simulink model "power_KundurTwoAreaSystem"  (R2023a)
settings: Solver=FixedStepDiscrete  StartTime=0.0  StopTime=5  MaxStep=1/60  RelTol=1e-4
PreLoadFcn:
  | Ts=50e-6;
  | Tctrl=2*Ts;
  | PSSMODEL=1;
undefined symbols (not defined in the file): D1, Delta
libraries: spsThreePhaseVIMeasurementLib x15, spsGenericPowerSystemStabilizerLib x8, spsLoadFlowBusLib x6, spsThreePhaseParallelRLCLoadLib x4, spsThreePhasePISectionLineLib x4, spsSynchronousMachinepuStandardLib x4, spsExcitationSystemLib x4, spsSteamTurbineandGovernorLib x4, spsThreePhaseSeriesRLCLoadLib x4, spsThreePhaseTransformerTwoWindingsLib x4, spsThreePhaseFaultLib x4, spsThreePhaseBreakerLib x2
(part 1 of 2)
settings Model: ARTEMISmethode_block_infos=$$__separator__$$  ExtModeTrigMode=oneshot  Creator=The MathWorks, Inc.  LastModifiedBy=LENOVO
settings SolverCC: AlgebraicLoopSolver=TrustRegion
settings DataIOCC: SaveOutput=off  SignalLogging=off  DSMLogging=off  SaveTime=off  ReturnWorkspaceOutputs=off  TimeSaveName=t  SignalLoggingName=sigsOut
settings OptimizationCC: BlockReduction=off  BooleanDataType=off  OptimizeBlockIOStorage=off  BufferReuse=off  ReuseModelBlockBuffer=off  GlobalBufferReuse=off  ExpressionFolding=off  ExpressionDepthLimit=2147483647  LocalBlockOutputs=off  InitFltsAndDblsToZero=on  LifeSpan=inf  OptimizeDataStoreBuffers=off  BusAssignmentInplaceUpdate=off
settings DebuggingCC: SaveWithParameterizedLinksMsg=none  SignalResolutionControl=TryResolveAllWithWarning  MultiTaskDSMMsg=warning  MultiTaskCondExecSysMsg=none  FcnCallInpInsideContextMsg=warning  UnconnectedInputMsg=warning  UnconnectedLineMsg=warning  StateNameClashWarn=warning  SFUnexpectedBacktrackingDiag=warning  SFNoUnconditionalDefaultTransitionDiag=warning  SFExecutionAtInitializationDiag=none  ArithmeticOperatorsInVariantConditions=warning
settings HardwareCC: ProdBitPerPointer=32  ProdBitPerSizeT=32  ProdBitPerPtrDiffT=32  ProdLargestAtomicFloat=None  ProdIntDivRoundTo=Undefined  ProdEndianess=Unspecified  ProdWordSize=32  ProdHWDeviceType=32-bit Generic  TargetBitPerPointer=64  TargetBitPerSizeT=64  TargetBitPerPtrDiffT=64  TargetLongLongMode=on  TargetIntDivRoundTo=Zero  TargetEndianess=LittleEndian  TargetWordSize=64  TargetHWDeviceType=MATLAB Host  ProdEqTarget=off
settings ModelReferenceCC: EnableRefExpFcnMdlSchedulingChecks=on  PropagateSignalLabelsOutOfModel=off
settings SFSimCC: SimUseLocalCustomCode=off  CustomCodeUndefinedFunction=UseInterfaceOnly
settings RTWCC: RTWUseLocalCustomCode=off
settings CodeAppCC: StateflowObjectComments=on
settings GRTTargetCC: TargetFcnLib=ansi_tfl_tmw.mat  TargetLangStandard=C89/C90 (ANSI)  CombineOutputUpdateFcns=off  GRTInterface=on
settings ConfigComp: CovMetricSettings=dw  CovSaveCumulativeToWorkspaceVar=on  CovSaveSingleToWorkspaceVar=on  CovExternalEMLEnable=off  CovSFcnEnable=off
settings SimscapeCC: SimscapeNormalizeSystem=off  SimscapeNominalValues={1, 'bar'; 1, 'cm^3/s'; 1, 'bar*kg/s'; 1, 'kJ/kg'; 1, 'kW'; }

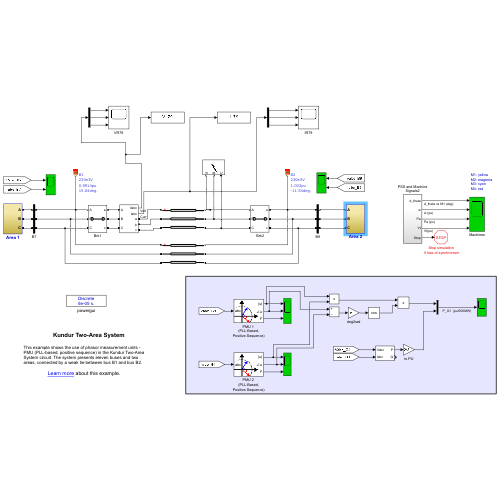
[thumbnail: Simulink's stored preview of the top-level diagram]
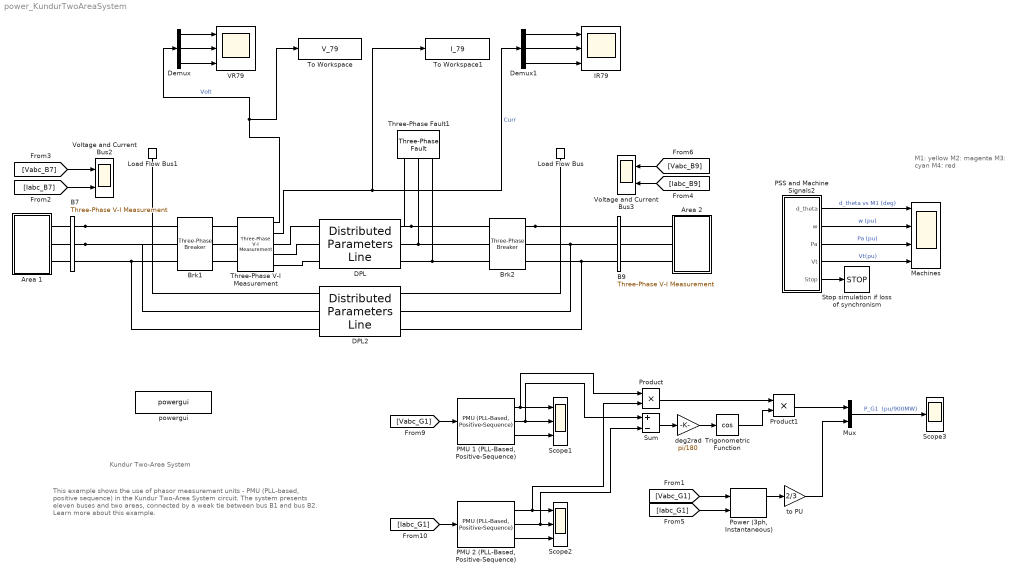
== system power_KundurTwoAreaSystem ==
  note: This example shows the use of phasor measurement units - PMU (PLL-based, positive sequence) in the Kundur Two-Area System circuit. The system presents eleven buses and two areas, connected by a weak tie between bus B1 and bus B2.
      |
      | Learn more about this example.
  note: M1: yellow
      | M2: magenta
      | M3: cyan
      | M4: red
  note: Kundur Two-Area System
  " Brk2" : spsThreePhaseBreakerLib/Three-Phase Breaker  InitialState=closed  SwitchA=on  SwitchB=on  SwitchC=on  SwitchTimes=[2+12]*100  External=off  BreakerResistance=0.001  SnubberResistance=1e6  SnubberCapacitance=0  Measurements=None
      settings: AttributesFormatString=\n
  Area 1 : Subsystem
  Area 2 : Subsystem
  B7 : spsThreePhaseVIMeasurementLib/Three-Phase V-I Measurement  VoltageMeasurement=phase-to-ground  SetLabelV=on  LabelV=Vabc_B7  Vpu=on  VpuLL=off  CurrentMeasurement=yes  SetLabelI=on  LabelI=Iabc_B7  Ipu=off  Pbase=100e6  Vbase=230e3  OutputType=Complex  PhasorSimulation=off  PSBequivalent=0
  B9 : spsThreePhaseVIMeasurementLib/Three-Phase V-I Measurement  VoltageMeasurement=phase-to-ground  SetLabelV=on  LabelV=Vabc_B9  Vpu=off  VpuLL=off  CurrentMeasurement=yes  SetLabelI=on  LabelI=Iabc_B9  Ipu=off  Pbase=100e6  Vbase=500e3  OutputType=Complex  PhasorSimulation=off  PSBequivalent=0
  Brk1 : spsThreePhaseBreakerLib/Three-Phase Breaker  InitialState=closed  SwitchA=off  SwitchB=off  SwitchC=off  SwitchTimes=[2+12]  External=off  BreakerResistance=0.001  SnubberResistance=inf  SnubberCapacitance=0  Measurements=None
      settings: AttributesFormatString=\n
  DPL : spsDistributedParametersLineLib/Distributed Parameters Line  Phases=3  Length=220  Frequency=60  Resistance=[0.0001*529 1.61]  Inductance=[0.001*529/(377) 0.0061]  Capacitance=[0.00175/529/(377) 5.2489e-9]  x1=[-0.00125 5.00367371114962e-05 67714.6934397594 -217896.109792038;-0.0012 4.86621318433669e-05 71809.6791282428 -216581.073841555;-0.00115 4.72702371515041e-05 75879.1511796623 -215189.087666813;-0.0011 4.58615475694642e-05 79921.6637299751 -213720.64583387;-0.00105 4.4436563597948e-05 83935.7804937212 -212176.270073119;-0.001 4.29957915269754e-05 87920.075274328 -210556.509093914;-0.00095 4.15397432560028e-05 91873.1324708315 -208861.938389617;-0.0009 4.00689361120477e-05 95793.547580833 -207093.160033131;-0.00085 3.8583892665885e-05 99679.9276995113 -205250.802462984;-0.0008 3.70851405463799e-05 103530.892014516 -203335.520260047;-0.00075 3.55732122530239e-05 107345.072296562 -201347.993914968;-0.0007 3.40486449667404e-05 111121.113385557 -199288.929586394;-0.00065 3.2511980359027e-05 114857.673672083 -197159.058850075;-0.0006 3.09637643995015e-05 118553.425574062 -194959.138438943;-0.00055 2.94045471619226e-05 122207.05600844 -192689.949974244;-0.0005 2.78348826287503e-05 125817.266857722 -190352.299687836;-0.00045 2.6255328494319e-05 129382.775431183 -187947.018135733;-0.0004 2.46664459666915e-05 132902.314920604 -185474.959903019;-0.00035 2.30687995682643e-05 136374.634850364 -182937.003300212;-0.0003 2.14629569351953e-05 139798.501521726 -180334.050051208;-0.00025 1.98494886157256e-05 143172.698451165 -177667.024972904;-0.0002 1.82289678674665e-05 146496.026802577 -174936.875646609;-0.00015 1.66019704537234e-05 149767.305813225 -172144.572081379;-0.0001 1.49690744389303e-05 152985.373213251 -169291.106369375;-5e-05 1.33308599832661e-05 156149.085638633 -166377.492333378]  x2=[-0.00125 6.6417563157089e-05 -37052.7419451155 -227701.023522909;-0.0012 6.59388164154627e-05 -32754.3455922343 -228358.945598922;-0.00115 6.54366419263393e-05 -28444.3117763279 -228935.732828921;-0.0011 6.49112181099238e-05 -24124.1718318883 -229431.180283151;-0.00105 6.43627316467963e-05 -19795.460684067 -229845.11193149;-0.001 6.37913774115854e-05 -15459.716303323 -230177.380705994;-0.00095 6.31973584037304e-05 -11118.4791589897 -230427.86855315;-0.0009 6.25808856753561e-05 -6773.29167195314 -230596.486475819;-0.00085 6.19421782562878e-05 -2425.69766663739 -230683.174564855;-0.0008 6.12814630762299e-05 1922.75817750908 -230687.902020394;-0.00075 6.059897488414e-05 6270.5308748305 -230610.667162792;-0.0007 5.98949561648229e-05 10616.07568239 -230451.497433227;-0.00065 5.91696570527773e-05 14957.8486488092 -230210.449383946;-0.0006 5.84233352433242e-05 19294.3071628271 -229887.608658174;-0.00055 5.76562559010488e-05 23623.9105013821 -229483.089959682;-0.0005 5.68686915655888e-05 27945.120377024 -228997.037012038;-0.00045 5.60609220548025e-05 32256.40148446 -228429.62250754;-0.0004 5.52332343653508e-05 36556.2220460412 -227781.04804586;-0.00035 5.43859225707287e-05 40843.0543559962 -227051.544062416;-0.0003 5.35192877167822e-05 45115.3753232175 -226241.369746499;-0.00025 5.26336377147484e-05 49371.6670124087 -225350.812949186;-0.0002 5.17292872318557e-05 53610.4171833994 -224380.190081066;-0.00015 5.08065575795247e-05 57830.1198284372 -223329.845999824;-0.0001 4.98657765992071e-05 62029.2757072648 -222200.153887709;-5e-05 4.89072785459056e-05 66206.3928797934 -220991.51511895]  x3=[-0.00125 5.67524045659529e-09 -83.9619667865334 325.434737438529;-0.0012 5.93441221514109e-09 -90.0809906089823 323.794335553023;-0.00115 6.19147550528425e-09 -96.1680090843992 322.03889108188;-0.0011 6.44633899366183e-09 -102.220859524104 320.169027726161;-0.00105 6.69891212848996e-09 -108.237391379156 318.185409839415;-0.001 6.9491051717365e-09 -114.215467004436 316.088742191629;-0.00095 7.19682923100451e-09 -120.15296241814 313.879769718837;-0.0009 7.44199629111529e-09 -126.04776805642 311.559277258439;-0.00085 7.68451924537978e-09 -131.8977895229 309.128089270358;-0.0008 7.92431192654714e-09 -137.70094833281 306.587069544109;-0.00075 8.16128913741954e-09 -143.455182651456 303.937120891901;-0.0007 8.39536668112235e-09 -149.158448026785 301.179184827873;-0.00065 8.6264613910189e-09 -154.808718115766 298.314241233575;-0.0006 8.85449116025912e-09 -160.40398540434 295.343308009826;-0.00055 9.07937497095181e-09 -165.942261920683 292.267440715053;-0.0005 9.30103292294984e-09 -171.421579941519 289.08773219026;-0.00045 9.51938626223831e-09 -176.839992691245 285.805312170745;-0.0004 9.73435740891549e-09 -182.195575033613 282.421346884711;-0.00035 9.94586998475657e-09 -187.486424155717 278.937038638912;-0.0003 1.01538488403505e-08 -192.710660244058 275.353625391476;-0.00025 1.03582200818002e-08 -197.866427152428 271.672380312068;-0.0002 1.05589110969767e-08 -202.951893061395 267.894611329534;-0.00015 1.0755850581318e-08 -207.965251129137 264.021660667207;-0.0001 1.0948968563163e-08 -212.904720133404 260.054904366015;-5e-05 1.11381964286123e-08 -217.768545104379 255.995751795585]  x4=[-0.00125 9.68464422615185e-08 -1.96836906133708 -1426.6168237965;-0.0012 9.56560270886339e-08 24.921520258627 -1426.40038533004;-0.00115 9.44316257848021e-08 51.80255508111 -1425.67715359865;-0.0011 9.31736733739763e-08 78.6651847024365 -1424.44738556312;-0.00105 9.18826168006582e-08 105.499864958212 -1422.71151815417;-0.001 9.05589147711008e-08 132.297061614318 -1420.47016811722;-0.00095 8.92030375903321e-08 159.04725375438 -1417.72413179328;-0.0009 8.78154669950584e-08 185.740937162506 -1414.47438483598;-0.00085 8.63966959825051e-08 212.368627700085 -1410.72208186493;-0.0008 8.49472286352572e-08 238.920864675461 -1406.46855605551;-0.00075 8.34675799421615e-08 265.388214205267 -1401.7153186652;-0.0007 8.19582756153531e-08 291.761272566243 -1396.46405849659;-0.00065 8.04198519034725e-08 318.030669536333 -1390.71664129743;-0.0006 7.88528554011392e-08 344.187071723876 -1384.47510909768;-0.00055 7.72578428547491e-08 370.221185883724 -1377.741679484;-0.0005 7.56353809646651e-08 396.123762219079 -1370.51874481189;-0.00045 7.39860461838711e-08 421.885597667908 -1362.80887135563;-0.0004 7.23104245131612e-08 447.497539172743 -1354.61479839655;-0.00035 7.06091112929365e-08 472.950486932723 -1345.93943724976;-0.0003 6.88827109916829e-08 498.235397636705 -1336.78587022977;-0.00025 6.71318369912072e-08 523.343287676313 -1327.15734955535;-0.0002 6.53571113687047e-08 548.26523633777 -1317.05729619404;-0.00015 6.35591646757385e-08 572.992388971387 -1306.48929864672;-0.0001 6.17386357142074e-08 597.515960137573 -1295.4571116726;-5e-05 5.98961713093829e-08 621.827236728265 -1283.96465495517]  x5=0.00124486354111605  V1=ones(3,3)  V2=ones(3,3)  I1=ones(3,3)  I2=ones(3,3)  nHarmo=1  Measurements=None  Decoupling=off  VsMag0=0  VrMag0=0  VsAngle0=0  VrAngle0=0  IsMag0=0  IrMag0=0  IsAngle0=0  IrAngle0=0
      settings: LibrarySourceBlock=sps_lib/Power Grid Elements/Distributed Parameters Line
  DPL2 : spsDistributedParametersLineLib/Distributed Parameters Line  Phases=3  Length=220  Frequency=60  Resistance=[0.0001*529 1.61]  Inductance=[0.001*529/(377) 0.0061]  Capacitance=[0.00175/529/(377) 5.2489e-9]  x1=[-0.00125 5.00379847973649e-05 67714.9467441329 -217896.980956182;-0.0012 4.86633839020789e-05 71809.9488077379 -216581.940076482;-0.00115 4.72714931382089e-05 75879.437138463 -215189.948664753;-0.0011 4.58628070379157e-05 79921.9658664817 -213721.501288916;-0.00105 4.44378261006631e-05 83936.098700586 -212177.119681331;-0.001 4.29970566153929e-05 87920.4094384935 -210557.352553429;-0.00095 4.15410104806428e-05 91873.4824735709 -208862.775400759;-0.0009 4.00702050226714e-05 95793.913297792 -207093.990298514;-0.00085 3.85851628116544e-05 99680.3090007523 -205251.625687619;-0.0008 3.70864114760182e-05 103531.288764564 -203336.336151446;-0.00075 3.5574483514976e-05 107345.484354455 -201348.802183249;-0.0007 3.40499161093329e-05 111121.540604892 -199289.729944382;-0.00065 3.25132509306289e-05 114858.115901071 -197159.851013407;-0.0006 3.0965033948685e-05 118553.88265558 -194959.922126168;-0.00055 2.94058152376227e-05 122207.527780091 -192690.724906921;-0.0005 2.78361487804258e-05 125817.753151886 -190353.065590635;-0.00045 2.62565922721123e-05 129383.276075083 -187947.774736533;-0.0004 2.46677069215884e-05 132902.829736365 -185475.706933003;-0.00035 2.30700572522534e-05 136375.163655073 -182937.740493963;-0.0003 2.14642109014275e-05 139799.044127501 -180334.777146806;-0.00025 1.98507384186727e-05 143173.25466522 -177667.741712014;-0.0002 1.82302130630794e-05 146496.596427293 -174937.581774578;-0.00015 1.66032105995901e-05 149767.888646217 -172145.267347323;-0.0001 1.49703090944329e-05 152985.969047441 -169291.790526269;-5e-05 1.33320887097373e-05 156149.694262324 -166378.165138145]  x2=[-0.00125 6.64176958426058e-05 -37052.8319738182 -227700.14152326;-0.0012 6.59389266485741e-05 -32754.4522292874 -228358.065452929;-0.00115 6.54367296678802e-05 -28444.4349838437 -228934.854849298;-0.0011 6.49112833287199e-05 -24124.3115660918 -229430.304781838;-0.00105 6.43627743196758e-05 -19795.6168953113 -229844.239219549;-0.001 6.37913975233868e-05 -15459.888936107 -230176.511093496;-0.00095 6.3197355947308e-05 -11118.6681519778 -230427.002349064;-0.0009 6.25808606515828e-05 -6773.496957997 -230595.623987903;-0.00085 6.19421306740542e-05 -2425.91917279987 -230682.316099547;-0.0008 6.12813929524419e-05 1922.52052992806 -230687.047882702;-0.00075 6.05988822437122e-05 6270.277170266 -230609.817656188;-0.0007 5.98948410406701e-05 10615.806010982 -230450.652859537;-0.00065 5.91695194858025e-05 14957.5631063708 -230209.610043242;-0.0006 5.84231752824043e-05 19294.00585081 -229886.77484867;-0.00055 5.76560736030171e-05 23623.5935268411 -229482.261977626;-0.0005 5.68684869952149e-05 27944.7878525787 -228996.215151609;-0.00045 5.60606952847694e-05 32256.0535282547 -228428.807060741;-0.0004 5.52329854762288e-05 36555.8587817031 -227780.239302415;-0.00035 5.43856516509468e-05 40842.6759125913 -227050.742309668;-0.0003 5.3518994862597e-05 45114.9818352051 -226240.575269306;-0.00025 5.26333230302095e-05 49371.2586195931 -225350.026029823;-0.0002 5.17289508287692e-05 53609.9940308807 -224379.410999122;-0.00015 5.08061995774129e-05 57829.6820665593 -223329.075032102;-0.0001 4.98653971252664e-05 62028.8234915626 -222199.391308131;-5e-05 4.89068777349613e-05 66205.9263709369 -220990.761198457]  x3=[-0.00125 5.67701476718236e-09 -83.9470362519072 325.436899755658;-0.0012 5.93614409507095e-09 -90.0661034818627 323.796778902833;-0.00115 6.19316433922822e-09 -96.1531706541115 322.04161459626;-0.0011 6.44798418158524e-09 -102.206075062672 320.17203043746;-0.00105 6.70051308586539e-09 -108.222666139428 318.188690680783;-0.001 6.95066132975141e-09 -114.20080621822 316.0922999974;-0.00095 7.19834003676336e-09 -120.138371294344 313.883603224938;-0.0009 7.443461207836e-09 -126.0332517792 311.563385102845;-0.00085 7.68593775258441e-09 -131.88335324982 309.13246999357;-0.0008 7.92568352024683e-09 -137.686597193009 306.591721589677;-0.00075 8.16261333029358e-09 -143.440921743827 303.942042606977;-0.0007 8.39664300269133e-09 -149.14428241816 301.184374463793;-0.00065 8.62768938781182e-09 -154.794652839118 298.319696946488;-0.0006 8.85567039597459e-09 -160.390025456994 295.349027861342;-0.00055 9.08050502661299e-09 -165.928412262543 292.273422672937;-0.0005 9.30211339705333e-09 -171.407845493302 289.09397412915;-0.00045 9.5204167708968e-09 -176.826378332736 285.81181187291;-0.0004 9.73533758599417e-09 -182.182085601928 282.428102040838;-0.00035 9.94679948200319e-09 -187.473064443587 278.944046848926;-0.0003 1.01547273275191e-08 -192.697434998124 275.360884165393;-0.00025 1.03590472467685e-08 -197.853341071558 271.67988707088;-0.0002 1.05596866458569e-08 -202.938950795012 267.902363406126;-0.00015 1.07565742385613e-08 -207.952457275566 264.029655307303;-0.0001 1.09496400716574e-08 -212.89207923824 260.063138729157;-5e-05 1.1138815549774e-08 -217.756061658871 256.004222956143]  x4=[-0.00125 9.68461057473568e-08 -1.98289624558899 -1426.61901857765;-0.0012 9.56557230997411e-08 24.9070370221481 -1426.40285353559;-0.00115 9.44313544291841e-08 51.788120938229 -1425.67989435166;-0.0011 9.31734347480444e-08 78.6508047815356 -1424.45039788981;-0.00105 9.1882410989195e-08 105.485544368409 -1422.71480098428;-0.001 9.05587418472302e-08 132.282805443649 -1420.47372028438;-0.00095 8.92028976154931e-08 159.033067067996 -1417.72795203541;-0.0009 8.78153600189834e-08 185.726825000868 -1414.47847179577;-0.00085 8.63966220432021e-08 212.354595077178 -1410.72643409031;-0.0008 8.49471877589966e-08 238.906916577008 -1406.47317200015;-0.00075 8.34675721434664e-08 265.374355586962 -1401.72019668907;-0.0007 8.19583008969943e-08 291.747508351987 -1396.46919686656;-0.00065 8.04199102564676e-08 318.017004616485 -1390.72203818786;-0.0006 7.88529468047557e-08 344.173510953518 -1384.48076259108;-0.00055 7.72579672765117e-08 370.207734080932 -1377.74758757171;-0.0005 7.56355383603673e-08 396.110424163215 -1370.5249053948;-0.00045 7.3986236497591e-08 421.872378097919 -1362.81528224491;-0.0004 7.23106476772813e-08 447.484442785481 -1354.62145731444;-0.00035 7.06093672281675e-08 472.93751838127 -1345.94634183038;-0.0003 6.88829996070924e-08 498.222561528727 -1336.79301801995;-0.00025 6.71321581842514e-08 523.330588572417 -1327.16473801552;-0.0002 6.53574650252652e-08 548.252678749889 -1317.06492269912;-0.00015 6.35595506701629e-08 572.97997736117 -1306.49716048704;-0.0001 6.17390539093537e-08 597.503698914807 -1295.46520605489;-5e-05 5.98966215566684e-08 621.815130249304 -1283.97297900353]  x5=0.00124486354111605  V1=ones(3,3)  V2=ones(3,3)  I1=ones(3,3)  I2=ones(3,3)  nHarmo=1  Measurements=None  Decoupling=off  VsMag0=0  VrMag0=0  VsAngle0=0  VrAngle0=0  IsMag0=0  IrMag0=0  IsAngle0=0  IrAngle0=0
      settings: LibrarySourceBlock=sps_lib/Power Grid Elements/Distributed Parameters Line
  Demux : Demux  Outputs=3
  Demux1 : Demux  Outputs=3
  IR79 : Scope  NumInputPorts=3
  Load Flow Bus : spsLoadFlowBusLib/Load Flow Bus  LConnTagsString=a  Phases=single  Connectors=on one side  ID=B2  Vbase=230e3  Vref=1  Vangle=0  VLF=1.003  VLFb=1  VLFc=1  angleLF=-11.54  angleLFb=0  angleLFc=0
      settings: AttributesFormatString=%<ID>\n%<Vbase>V\n%<VLF>pu\n%<angleLF>deg.
  Load Flow Bus1 : spsLoadFlowBusLib/Load Flow Bus  LConnTagsString=a  Phases=single  Connectors=on one side  ID=B1  Vbase=230e3  Vref=1  Vangle=0  VLF=0.9914  VLFb=1  VLFc=1  angleLF=15.04  angleLFb=0  angleLFc=0
      settings: AttributesFormatString=%<ID>\n%<Vbase>V\n%<VLF>pu\n%<angleLF>deg.
  Machines : Scope  NumInputPorts=4
  Mux : Mux  Inputs=2
  "PMU 1 (PLL-Based, Positive-Sequence)" : spsPMUPLLBasedPositiveSequenceLib/PMU (PLL-Based, Positive-Sequence)  nominalFrequency=60  samplingRate=64  reportingFactor=1
      settings: LibrarySourceBlock=|
      | sps_lib/Sensors and Measurements/PMU
      | (PLL-Based,
      | Positive-Sequence)
  "PMU 2 (PLL-Based, Positive-Sequence)" : spsPMUPLLBasedPositiveSequenceLib/PMU (PLL-Based, Positive-Sequence)  nominalFrequency=60  samplingRate=64  reportingFactor=1
      settings: LibrarySourceBlock=|
      | sps_lib/Sensors and Measurements/PMU
      | (PLL-Based,
      | Positive-Sequence)
  PSS and Machine Signals2 : Subsystem
  "Power (3ph, Instantaneous)" : spsPower3phInstantaneousLib/Power (3ph, Instantaneous)
  Product : Product
  Product1 : Product
  Scope1 : Scope  NumInputPorts=3
  Scope2 : Scope  NumInputPorts=3
  Scope3 : Scope
  Stop simulation if loss of synchronism : Stop
  Sum : Sum  Inputs=+-
  Three-Phase V-I Measurement : spsThreePhaseVIMeasurementLib/Three-Phase V-I Measurement  VoltageMeasurement=phase-to-ground  SetLabelV=off  LabelV=Vabc  Vpu=off  VpuLL=off  CurrentMeasurement=yes  SetLabelI=off  LabelI=Iabc  Ipu=off  Pbase=100e6  Vbase=500e3  OutputType=Complex  PhasorSimulation=off  PSBequivalent=0
  Three-Phase Fault1 : spsThreePhaseFaultLib/Three-Phase Fault  InitialStates=0  FaultA=off  FaultB=off  FaultC=off  GroundFault=off  SwitchTimes=[0 0.1]  External=off  SwitchStatus=NaN  FaultResistance=0.001  GroundResistance=0.001  SnubberResistance=1e6  SnubberCapacitance=inf  Measurements=None
  To Workspace : ToWorkspace  VariableName=V_79  SampleTime=0.01
  To Workspace1 : ToWorkspace  VariableName=I_79  SampleTime=0.01
  Trigonometric Function : Trigonometry  Operator=cos
  VR79 : Scope  NumInputPorts=3
  Voltage and Current Bus2 : Scope  NumInputPorts=2
  Voltage and Current Bus3 : Scope  NumInputPorts=2
  deg2rad : Gain  Gain=pi/180
  powergui : spspowerguiLib/powergui  Priority=2  SimulationMode=Discrete  SampleTime=Ts  frequency=60  Iterations=50  frequencyindice=0  Pbase=100e6  ErrMax=1e-4  UnitsV=kV  UnitsW=MW  buscounter=0  FunctionMessages=off  echomessages=off  EnableUseOfTLC=off  CurrentSourceSwitches=off  DisableSnubberDevices=off  DisableRonSwitches=off  DisableVfSwitches=off  DisplayEquations=off  AutomaticDiscreteSolvers=off  SolverType=Tustin  Interpol=off  ExternalGateDelay=off  methode=off  Ts=0  x0status=blocks  SPID=off  SwTol=0  HookPort=off  NonlinearTolerance=1e-4  nMaxIteration=100  ContinueOnMaxIteration=off  RestoreLinks=warning  ResistiveCurrentMeasurement=off  Frange=logspace(0,3,50)  Ylog=off  Xlog=off  ShowGrid=off  save=off  variable=ZData  structure=0  ZoomFFT=on  StartTime=0.0  cycles=1  DisplayStyle=1  fundamental=60  FreqAxis=off  MaxFrequency=1000  frequencyindicesteady=1  RmsSteady=1  display=off
  to PU : Gain  Gain=2/3
  wires:
  [Iabc_B7] -> Voltage and Current Bus2/2
  [Vabc_B7] -> Voltage and Current Bus2/1
  [Iabc_B9] -> Voltage and Current Bus3/2
  [Vabc_B9] -> Voltage and Current Bus3/1
  PSS and Machine Signals2/1(d_theta) -> Machines/1  "d_theta vs M1 (deg)"
  PSS and Machine Signals2/2(w) -> Machines/2  "w (pu)"
  PSS and Machine Signals2/3(Pa) -> Machines/3  "Pa (pu)"
  PSS and Machine Signals2/4(Vt) -> Machines/4  "Vt(pu)"
  PSS and Machine Signals2/5(Stop) -> Stop simulation if loss of synchronism/1
  [Iabc_G1] -> "PMU 2 (PLL-Based, Positive-Sequence)"/1
  "PMU 2 (PLL-Based, Positive-Sequence)"/3 -> Scope2/3
  [Vabc_G1] -> "PMU 1 (PLL-Based, Positive-Sequence)"/1
  "PMU 1 (PLL-Based, Positive-Sequence)"/3 -> Scope1/3
  Product/1 -> Product1/1
  [Iabc_G1] -> "Power (3ph, Instantaneous)"/2
  "Power (3ph, Instantaneous)"/1 -> to PU/1
  "PMU 2 (PLL-Based, Positive-Sequence)"/1 -> Product/2, Scope2/1
  [Vabc_G1] -> "Power (3ph, Instantaneous)"/1
  "PMU 2 (PLL-Based, Positive-Sequence)"/2 -> Sum/2, Scope2/2
  deg2rad/1 -> Trigonometric Function/1
  "PMU 1 (PLL-Based, Positive-Sequence)"/1 -> Scope1/1, Product/1
  Trigonometric Function/1 -> Product1/2
  Product1/1 -> Mux/1
  Sum/1 -> deg2rad/1
  to PU/1 -> Mux/2
  "PMU 1 (PLL-Based, Positive-Sequence)"/2 -> Sum/1, Scope1/2
  Mux/1 -> Scope3/1  "P_G1  (pu/900MW)"
  Three-Phase V-I Measurement/1 -> To Workspace/1, Demux/1  "Volt"
  Three-Phase V-I Measurement/2 -> To Workspace1/1, Demux1/1  "Curr"
  Demux/1 -> VR79/1
  Demux/2 -> VR79/2
  Demux/3 -> VR79/3
  Demux1/1 -> IR79/1
  Demux1/2 -> IR79/2
  Demux1/3 -> IR79/3
  connections:
  " Brk2"/RConn1 -- DPL2/RConn1 -- B9/LConn1 -- Load Flow Bus/LConn1
  " Brk2"/RConn2 -- DPL2/RConn2 -- B9/LConn2
  " Brk2"/RConn3 -- DPL2/RConn3 -- B9/LConn3
  B9/RConn3 -- Area 2/LConn3
  B9/RConn2 -- Area 2/LConn2
  Area 2/LConn1 -- B9/RConn1
  Area 1/RConn3 -- B7/LConn3
  Area 1/RConn2 -- B7/LConn2
  Area 1/RConn1 -- B7/LConn1
  " Brk2"/LConn3 -- Three-Phase Fault1/LConn3 -- DPL/RConn3
  " Brk2"/LConn2 -- Three-Phase Fault1/LConn2 -- DPL/RConn2
  DPL/RConn1 -- " Brk2"/LConn1 -- Three-Phase Fault1/LConn1
  DPL2/LConn3 -- B7/RConn3 -- Brk1/LConn3
  B7/RConn2 -- DPL2/LConn2 -- Brk1/LConn2
  B7/RConn1 -- DPL2/LConn1 -- Brk1/LConn1 -- Load Flow Bus1/LConn1
  Three-Phase V-I Measurement/LConn1 -- Brk1/RConn1
  Three-Phase V-I Measurement/LConn2 -- Brk1/RConn2
  Three-Phase V-I Measurement/LConn3 -- Brk1/RConn3
  DPL/LConn1 -- Three-Phase V-I Measurement/RConn1
  DPL/LConn2 -- Three-Phase V-I Measurement/RConn2
  DPL/LConn3 -- Three-Phase V-I Measurement/RConn3

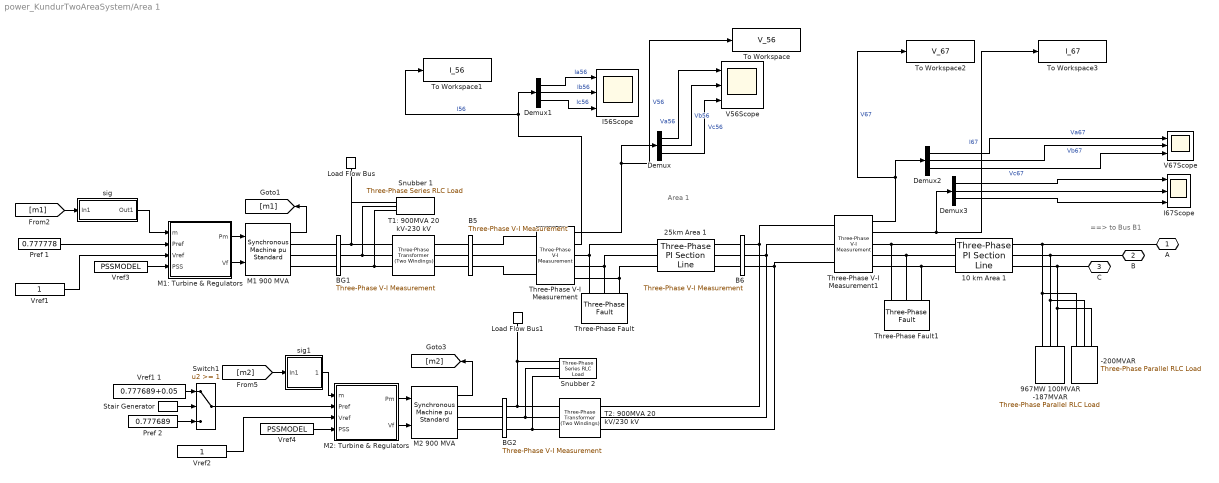
== system power_KundurTwoAreaSystem/Area 1 ==
  note: Area 1
  note: ==> to Bus B1
  -200MVAR : spsThreePhaseParallelRLCLoadLib/Three-Phase Parallel RLC Load  LConnTagsString=A|B|C  Configuration=Y (grounded)  NominalVoltage=230e3  Vabc=[1e3 1e3 1e3]  Vabcp=[1e3 1e3 1e3]  NominalFrequency=60  UnbalancedPower=off  ActivePower=0  InductivePower=0  CapacitivePower=200e6  Pabc=[10e3 9e3 11e3]  QLabc=[100 90 110]  QCabc=[100 90 110]  Pabcp=[10e3 9e3 11e3]  QLabcp=[100 90 110]  QCabcp=[100 90 110]  Measurements=None  LoadType=constant Z
  10 km Area 1 : spsThreePhasePISectionLineLib/Three-Phase PI Section Line  LConnTagsString=a|b|c  RConnTagsString=A|B|C  Length=10  Frequency=60  Resistances=[0.0001*529 1.61]  Inductances=[0.001*529/(377) 0.0061]  Capacitances=[0.00175/529/(377) 5.2489e-9]
  25km Area 1 : spsThreePhasePISectionLineLib/Three-Phase PI Section Line  LConnTagsString=a|b|c  RConnTagsString=A|B|C  Length=25  Frequency=60  Resistances=[0.0001*529 1.61]  Inductances=[0.001*529/(377) 0.0061]  Capacitances=[0.00175/529/(377) 5.2489e-9]
  967MW 100MVAR -187MVAR : spsThreePhaseParallelRLCLoadLib/Three-Phase Parallel RLC Load  LConnTagsString=A|B|C  Configuration=Y (grounded)  NominalVoltage=230e3  Vabc=[1e3 1e3 1e3]  Vabcp=[1e3 1e3 1e3]  NominalFrequency=60  UnbalancedPower=off  ActivePower=967e6  InductivePower=100e6  CapacitivePower=187e6  Pabc=[10e3 9e3 11e3]  QLabc=[100 90 110]  QCabc=[100 90 110]  Pabcp=[10e3 9e3 11e3]  QLabcp=[100 90 110]  QCabcp=[100 90 110]  Measurements=None  LoadType=constant Z
  B5 : spsThreePhaseVIMeasurementLib/Three-Phase V-I Measurement  VoltageMeasurement=phase-to-ground  SetLabelV=on  LabelV=Vabc_B5  Vpu=on  VpuLL=off  CurrentMeasurement=yes  SetLabelI=on  LabelI=Iabc_B5  Ipu=on  Pbase=900e6  Vbase=20e3  OutputType=Complex  PhasorSimulation=off  PSBequivalent=0
  B6 : spsThreePhaseVIMeasurementLib/Three-Phase V-I Measurement  VoltageMeasurement=phase-to-ground  SetLabelV=on  LabelV=Vabc_B6  Vpu=on  VpuLL=off  CurrentMeasurement=yes  SetLabelI=on  LabelI=Iabc_B6  Ipu=on  Pbase=900e6  Vbase=20e3  OutputType=Complex  PhasorSimulation=off  PSBequivalent=0
  BG1 : spsThreePhaseVIMeasurementLib/Three-Phase V-I Measurement  VoltageMeasurement=phase-to-ground  SetLabelV=on  LabelV=Vabc_G1  Vpu=on  VpuLL=off  CurrentMeasurement=yes  SetLabelI=on  LabelI=Iabc_G1  Ipu=on  Pbase=900e6  Vbase=20e3  OutputType=Complex  PhasorSimulation=off  PSBequivalent=0
  BG2 : spsThreePhaseVIMeasurementLib/Three-Phase V-I Measurement  VoltageMeasurement=no  SetLabelV=on  LabelV=Vabc_G2  Vpu=on  VpuLL=off  CurrentMeasurement=no  SetLabelI=on  LabelI=Iabc_G2  Ipu=on  Pbase=900e6  Vbase=20e3  OutputType=Complex  PhasorSimulation=off  PSBequivalent=0
  Demux{,1..3} (4 alike) : Demux  Outputs=3
  I56Scope : Scope  NumInputPorts=3
  I67Scope : Scope  NumInputPorts=3
  Load Flow Bus : spsLoadFlowBusLib/Load Flow Bus  LConnTagsString=a  Phases=single  Connectors=on one side  ID=M1_Area1  Vbase=20e3  Vref=1  Vangle=0  VLF=1  VLFb=1  VLFc=1  angleLF=10.19  angleLFb=0  angleLFc=0
      settings: AttributesFormatString=%<ID>\n%<Vbase>V\n%<VLF>pu\n%<angleLF>deg.
  Load Flow Bus1 : spsLoadFlowBusLib/Load Flow Bus  LConnTagsString=a  Phases=single  Connectors=on one side  ID=M2_Area1  Vbase=20e3  Vref=1  Vangle=0  VLF=1  VLFb=1  VLFc=1  angleLF=0  angleLFb=0  angleLFc=0
      settings: AttributesFormatString=%<ID>\n%<Vbase>V\n%<VLF>pu\n%<angleLF>deg.
  M1 900 MVA : spsSynchronousMachinepuStandardLib/Synchronous Machine pu Standard  PresetModel=No  MechanicalLoad=Mechanical power Pm  ShowDetailedParameters=on  RotorType=Round  Units=per unit standard parameters  MeasurementBus=off  NominalParameters="[900E6  20000   60 ]"  Reactances1=[1.8 .3 .25 1.7 .55 .25 .2]  Reactances2=[ 1.305, 0.296, 0.252, 0.474, 0.243, 0.18 ]  dAxisTimeConstants=Open-circuit  qAxisTimeConstants=Open-circuit  TimeConstants1=[]  TimeConstants2=[8 .03 .4 .05]  TimeConstants3=[]  TimeConstants4=[]  TimeConstants5=[ 1.01, 0.053, 0.1 ]  TimeConstants6=[]  TimeConstants7=[]  TimeConstants8=[]  StatorResistance=0.0025  Mechanical="[ 6.5 0  4]"  PolePairs=4  InitialConditions=[0 -31.4247 0.784453 0.784453 0.784453 2.7401 -117.26 122.74 1.83395]  SetSaturation=off  Saturation=[0.6404,0.7127,0.8441,0.9214,0.9956,1.082,1.19,1.316,1.457;0.7,0.7698,0.8872,0.9466,0.9969,1.046,1.1,1.151,1.201]  LoadFlowParameters=[1 700000000 0 0 0]  TsPowergui=0  TsBlock=-1  IterativeModel=Trapezoidal non iterative  IterativeDiscreteModel=Trapezoidal non iterative  BusType=PV  Pref=700000000  Qref=0  Qmin=-inf  Qmax=inf  PLF=0  QLF=0
  M1: Turbine & Regulators : Subsystem
  M2 900 MVA : spsSynchronousMachinepuStandardLib/Synchronous Machine pu Standard  PresetModel=No  MechanicalLoad=Mechanical power Pm  ShowDetailedParameters=on  RotorType=Round  Units=per unit standard parameters  MeasurementBus=off  NominalParameters="[900E6  20000   60 ]"  Reactances1=[1.8 .3 .25 1.7 .55 .25 .2]  Reactances2=[ 1.305, 0.296, 0.252, 0.474, 0.243, 0.18 ]  dAxisTimeConstants=Open-circuit  qAxisTimeConstants=Open-circuit  TimeConstants1=[]  TimeConstants2=[8 .03 .4 .05]  TimeConstants3=[]  TimeConstants4=[]  TimeConstants5=[ 1.01, 0.053, 0.1 ]  TimeConstants6=[]  TimeConstants7=[]  TimeConstants8=[]  StatorResistance=0.0025  Mechanical="[ 6.5 0  4]"  PolePairs=4  InitialConditions=[0 -42.8075 0.788608 0.788608 0.788608 -9.54571 -129.546 110.454 1.86756]  SetSaturation=off  Saturation=[0.6404,0.7127,0.8441,0.9214,0.9956,1.082,1.19,1.316,1.457;0.7,0.7698,0.8872,0.9466,0.9969,1.046,1.1,1.151,1.201]  LoadFlowParameters=[2 700000000 0 0 0]  TsPowergui=0  TsBlock=-1  IterativeModel=Trapezoidal non iterative  IterativeDiscreteModel=Trapezoidal non iterative  BusType=swing  Pref=0  Qref=0  Qmin=-inf  Qmax=inf  PLF=0  QLF=0
  M2: Turbine & Regulators : Subsystem
  Pref 1 : Constant  Value=0.777778
  Pref 2 : Constant  Value=0.777689
  Snubber 1 : spsThreePhaseSeriesRLCLoadLib/Three-Phase Series RLC Load  LConnTagsString=A|B|C  Configuration=Y (grounded)  NominalVoltage=20000  Vabc=[1e3 1e3 1e3]  Vabcp=[1e3 1e3 1e3]  NominalFrequency=60  UnbalancedPower=off  ActivePower=1e6  InductivePower=0  CapacitivePower=1e7  Pabc=[10e3 9e3 11e3]  QLabc=[100 90 110]  QCabc=[100 90 110]  Pabcp=[10e3 9e3 11e3]  QLabcp=[100 90 110]  QCabcp=[100 90 110]  Measurements=None  LoadType=constant Z
  Snubber 2 : spsThreePhaseSeriesRLCLoadLib/Three-Phase Series RLC Load  LConnTagsString=A|B|C  Configuration=Y (grounded)  NominalVoltage=20000  Vabc=[1e3 1e3 1e3]  Vabcp=[1e3 1e3 1e3]  NominalFrequency=60  UnbalancedPower=off  ActivePower=1e6  InductivePower=0  CapacitivePower=1e7  Pabc=[10e3 9e3 11e3]  QLabc=[100 90 110]  QCabc=[100 90 110]  Pabcp=[10e3 9e3 11e3]  QLabcp=[100 90 110]  QCabcp=[100 90 110]  Measurements=None  LoadType=constant Z
  Stair Generator : spsStairGeneratorLib/Stair Generator  t=[0 15 20]  e=[0 1 0 ]  Ts=0
  Switch1 : Switch  Threshold=1  SaturateOnIntegerOverflow=off
  T1: 900MVA 20 kV-230 kV : spsThreePhaseTransformerTwoWindingsLib/Three-Phase Transformer (Two Windings)  Winding1Connection=Delta (D1)  Winding2Connection=Yg  CoreType=Three single-phase transformers  SetSaturation=off  Hysteresis=off  DataFile='hysteresis'  SetInitialFlux=off  Measurements=None  UNITS=pu  NominalPower="[ 900e6   60 ]"  Winding1="[ 20e3  1e-6   0  ]"  Winding2="[ 230e3  1e-6   0.15 ]"  Rm=500  Lm=500  L0=0.5  Saturation="[ 0,0  ;  0.005,1.2  ;  1.0,1.4 ]"  InitialFluxes=[ 0.8 , -0.8 , 0.7 ]  BreakLoop=off  DiscreteSolver=Trapezoidal iterative  DataType=off  TransfoNumber=0
  T2: 900MVA 20 kV/230 kV : spsThreePhaseTransformerTwoWindingsLib/Three-Phase Transformer (Two Windings)  Winding1Connection=Delta (D1)  Winding2Connection=Yg  CoreType=Three single-phase transformers  SetSaturation=off  Hysteresis=off  DataFile='hysteresis'  SetInitialFlux=off  Measurements=None  UNITS=pu  NominalPower=[ 900e6 60 ]  Winding1="[ 20e3 1e-6  0.0]"  Winding2=[ 230e3 1e-6 0.15]  Rm=500  Lm=500  L0=0.5  Saturation="[ 0,0  ;  0.005,1.2  ;  1.0,1.4 ]"  InitialFluxes=[ 0.8 , -0.8 , 0.7 ]  BreakLoop=off  DiscreteSolver=Trapezoidal iterative  DataType=off  TransfoNumber=0
  Three-Phase V-I Measurement : spsThreePhaseVIMeasurementLib/Three-Phase V-I Measurement  VoltageMeasurement=phase-to-ground  SetLabelV=off  LabelV=Vabc  Vpu=off  VpuLL=off  CurrentMeasurement=yes  SetLabelI=off  LabelI=Iabc  Ipu=off  Pbase=100e6  Vbase=500e3  OutputType=Complex  PhasorSimulation=off  PSBequivalent=0
  Three-Phase V-I Measurement1 : spsThreePhaseVIMeasurementLib/Three-Phase V-I Measurement  VoltageMeasurement=phase-to-ground  SetLabelV=off  LabelV=Vabc  Vpu=off  VpuLL=off  CurrentMeasurement=yes  SetLabelI=off  LabelI=Iabc  Ipu=off  Pbase=100e6  Vbase=500e3  OutputType=Complex  PhasorSimulation=off  PSBequivalent=0
  Three-Phase Fault : spsThreePhaseFaultLib/Three-Phase Fault  InitialStates=0  FaultA=on  FaultB=off  FaultC=off  GroundFault=on  SwitchTimes=[2 2.1]  External=off  SwitchStatus=NaN  FaultResistance=0.001  GroundResistance=0.001  SnubberResistance=1e6  SnubberCapacitance=inf  Measurements=None
  Three-Phase Fault1 : spsThreePhaseFaultLib/Three-Phase Fault  InitialStates=0  FaultA=off  FaultB=off  FaultC=off  GroundFault=off  SwitchTimes=[0 0.1]  External=off  SwitchStatus=NaN  FaultResistance=0.001  GroundResistance=0.001  SnubberResistance=1e6  SnubberCapacitance=inf  Measurements=None
  To Workspace : ToWorkspace  VariableName=V_56  SampleTime=0.01
  To Workspace1 : ToWorkspace  VariableName=I_56  SampleTime=0.01
  To Workspace2 : ToWorkspace  VariableName=V_67  SampleTime=0.01
  To Workspace3 : ToWorkspace  VariableName=I_67  SampleTime=0.01
  V56Scope : Scope  NumInputPorts=3
  V67Scope : Scope  NumInputPorts=3
  Vref1 : Constant
  Vref1 1 : Constant  Value=0.777689+0.05
  Vref2 : Constant
  Vref3 : Constant  Value=PSSMODEL
  Vref4 : Constant  Value=PSSMODEL
  sig : Subsystem
  sig1 : Subsystem
  " A" : PMIOPort  Side=Right
  " B" : PMIOPort  Port=2  Side=Right
  " C" : PMIOPort  Port=3  Side=Right
  wires:
  Pref 1/1 -> M1: Turbine & Regulators/2(Pref)
  Vref2/1 -> M2: Turbine & Regulators/3(Vref)
  Vref4/1 -> M2: Turbine & Regulators/4(PSS)
  sig/1(Out1) -> M1: Turbine & Regulators/1(m)
  M1 900 MVA/1 -> [m1]
  M2 900 MVA/1 -> [m2]
  [m1] -> sig/1(In1)
  Vref3/1 -> M1: Turbine & Regulators/4(PSS)
  sig1/1(Out1) -> M2: Turbine & Regulators/1(m)
  [m2] -> sig1/1(In1)
  Stair Generator/1 -> Switch1/2
  Pref 2/1 -> Switch1/3
  Vref1 1/1 -> Switch1/1
  Switch1/1 -> M2: Turbine & Regulators/2(Pref)
  Vref1/1 -> M1: Turbine & Regulators/3(Vref)
  M1: Turbine & Regulators/1(Pm) -> M1 900 MVA/1
  M1: Turbine & Regulators/2(Vf) -> M1 900 MVA/2
  M2: Turbine & Regulators/2(Vf) -> M2 900 MVA/2
  M2: Turbine & Regulators/1(Pm) -> M2 900 MVA/1
  Three-Phase V-I Measurement/1 -> To Workspace/1, Demux/1  "V56"
  Demux/1 -> V56Scope/1  "Va56"
  Demux/2 -> V56Scope/2  "Vb56"
  Demux/3 -> V56Scope/3  "Vc56"
  Demux1/1 -> I56Scope/1  "Ia56"
  Demux1/3 -> I56Scope/3  "Ic56"
  Demux1/2 -> I56Scope/2  "Ib56"
  Three-Phase V-I Measurement/2 -> To Workspace1/1, Demux1/1  "I56"
  Three-Phase V-I Measurement1/1 -> To Workspace2/1, Demux2/1  "V67"
  Three-Phase V-I Measurement1/2 -> To Workspace3/1, Demux3/1  "I67"
  Demux2/1 -> V67Scope/1  "Va67"
  Demux2/2 -> V67Scope/2  "Vb67"
  Demux2/3 -> V67Scope/3  "Vc67"
  Demux3/1 -> I67Scope/1
  Demux3/2 -> I67Scope/2
  Demux3/3 -> I67Scope/3
  connections:
  Snubber 2/LConn1 -- T2: 900MVA 20 kV/230 kV/LConn1 -- BG2/RConn1 -- Load Flow Bus1/LConn1
  Snubber 2/LConn2 -- BG2/RConn2 -- T2: 900MVA 20 kV/230 kV/LConn2
  Snubber 2/LConn3 -- BG2/RConn3 -- T2: 900MVA 20 kV/230 kV/LConn3
  10 km Area 1/RConn1 -- " A"/RConn1 -- 967MW 100MVAR -187MVAR/LConn1 -- -200MVAR/LConn1
  10 km Area 1/RConn2 -- " B"/RConn1 -- 967MW 100MVAR -187MVAR/LConn2 -- -200MVAR/LConn2
  10 km Area 1/RConn3 -- " C"/RConn1 -- 967MW 100MVAR -187MVAR/LConn3 -- -200MVAR/LConn3
  Snubber 1/LConn1 -- Load Flow Bus/LConn1 -- BG1/RConn1 -- T1: 900MVA 20 kV-230 kV/LConn1
  T1: 900MVA 20 kV-230 kV/LConn2 -- BG1/RConn2 -- Snubber 1/LConn2
  T1: 900MVA 20 kV-230 kV/LConn3 -- BG1/RConn3 -- Snubber 1/LConn3
  Three-Phase V-I Measurement1/LConn2 -- B6/RConn2 -- T2: 900MVA 20 kV/230 kV/RConn2
  Three-Phase V-I Measurement1/LConn1 -- B6/RConn1 -- T2: 900MVA 20 kV/230 kV/RConn1
  Three-Phase V-I Measurement1/LConn3 -- B6/RConn3 -- T2: 900MVA 20 kV/230 kV/RConn3
  M1 900 MVA/RConn1 -- BG1/LConn1
  M1 900 MVA/RConn2 -- BG1/LConn2
  M1 900 MVA/RConn3 -- BG1/LConn3
  M2 900 MVA/RConn1 -- BG2/LConn1
  M2 900 MVA/RConn2 -- BG2/LConn2
  M2 900 MVA/RConn3 -- BG2/LConn3
  Three-Phase V-I Measurement/RConn1 -- 25km Area 1/LConn1 -- Three-Phase Fault/LConn1
  Three-Phase V-I Measurement/RConn2 -- 25km Area 1/LConn2 -- Three-Phase Fault/LConn2
  Three-Phase V-I Measurement/RConn3 -- 25km Area 1/LConn3 -- Three-Phase Fault/LConn3
  Three-Phase V-I Measurement1/RConn1 -- Three-Phase Fault1/LConn1 -- 10 km Area 1/LConn1
  Three-Phase V-I Measurement1/RConn2 -- Three-Phase Fault1/LConn2 -- 10 km Area 1/LConn2
  Three-Phase V-I Measurement1/RConn3 -- Three-Phase Fault1/LConn3 -- 10 km Area 1/LConn3
  B5/LConn1 -- T1: 900MVA 20 kV-230 kV/RConn1
  B5/LConn2 -- T1: 900MVA 20 kV-230 kV/RConn2
  B5/LConn3 -- T1: 900MVA 20 kV-230 kV/RConn3
  B5/RConn1 -- Three-Phase V-I Measurement/LConn1
  B5/RConn2 -- Three-Phase V-I Measurement/LConn2
  B5/RConn3 -- Three-Phase V-I Measurement/LConn3
  B6/LConn1 -- 25km Area 1/RConn1
  B6/LConn2 -- 25km Area 1/RConn2
  B6/LConn3 -- 25km Area 1/RConn3
